simulink model "simple"  (Simulink 7.3)
settings: Solver=ode45  StartTime=0.0  StopTime=200  RelTol=1e-3
libraries: truetime x1
settings Model: Creator=anton  LastModifiedBy=nmd01  ExtModeAutoUpdateStatusClock=off
settings OptimizationCC: BooleanDataType=off
settings DebuggingCC: SaveWithParameterizedLinksMsg=none  SignalResolutionControl=TryResolveAllWithWarning  SolverPrmCheckMsg=none  MultiTaskDSMMsg=warning  MultiTaskCondExecSysMsg=none  StrictBusMsg=None
settings HardwareCC: TargetUnknown=on
settings RTWCC: IncludeERTFirstTime=on

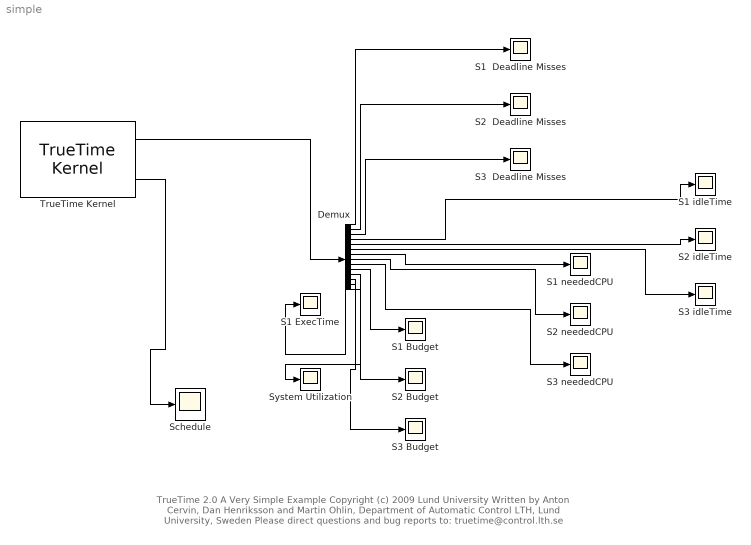
== system simple ==
  note: TrueTime 2.0  A Very Simple Example
      | Copyright (c) 2009 Lund University
      | Written by Anton Cervin, Dan Henriksson and Martin Ohlin,
      | Department of Automatic Control LTH, Lund University, Sweden
      | Please direct questions and bug reports to: truetime@control.lth.se
  Demux : Demux  Outputs=14
  S1 Budget : Scope
      settings: TimeRange=10  YMin=0  YMax=2  SaveName=ScopeData10
  S1 ExecTime : Scope
      settings: TimeRange=10  YMin=0  YMax=2  SaveName=ScopeData13
  S1 idleTime : Scope
      settings: TimeRange=10  YMin=0  YMax=2  SaveName=ScopeData4
  S1 neededCPU : Scope
      settings: TimeRange=10  YMin=0  YMax=2  SaveName=ScopeData7
  S1  Deadline Misses : Scope
      settings: TimeRange=10  YMin=0  YMax=2
  S2 Budget : Scope
      settings: TimeRange=10  YMin=0  YMax=2  SaveName=ScopeData11
  S2 idleTime : Scope
      settings: TimeRange=1000  YMin=0  YMax=0.35  SaveName=ScopeData5
  S2 neededCPU : Scope
      settings: TimeRange=10  YMin=0  YMax=2  SaveName=ScopeData8
  S2  Deadline Misses : Scope
      settings: TimeRange=10  YMin=0  YMax=2  SaveName=ScopeData2
  S3 Budget : Scope
      settings: TimeRange=10  YMin=0  YMax=2  SaveName=ScopeData12
  S3 idleTime : Scope
      settings: TimeRange=10  YMin=0  YMax=2  SaveName=ScopeData6
  S3 neededCPU : Scope
      settings: TimeRange=10  YMin=0  YMax=2  SaveName=ScopeData9
  S3  Deadline Misses : Scope
      settings: TimeRange=10  YMin=0  YMax=2  SaveName=ScopeData3
  Schedule : Scope
      settings: TimeRange=10  YMin=1  YMax=20
  System Utilization : Scope
      settings: TimeRange=10  YMin=0.945  YMax=1.06  SaveName=ScopeData14
  TrueTime Kernel : truetime/TrueTime Kernel  SystemSampleTime=-1  sfun=simple_init  args=[]  ninputsoutputs=[0 14]  ntriggers=0  trigtype=falling  nwnodenbr=[]  clockoffsetdrift=[0 0]  schedoutput=on  battery=off  poweroutput=off
  wires:
  TrueTime Kernel/2 -> Schedule/1
  TrueTime Kernel/1 -> Demux/1
  Demux/1 -> S1  Deadline Misses/1
  Demux/2 -> S2  Deadline Misses/1
  Demux/3 -> S3  Deadline Misses/1
  Demux/4 -> S1 idleTime/1
  Demux/5 -> S2 idleTime/1
  Demux/6 -> S3 idleTime/1
  Demux/7 -> S1 neededCPU/1
  Demux/8 -> S2 neededCPU/1
  Demux/9 -> S3 neededCPU/1
  Demux/10 -> S1 Budget/1
  Demux/11 -> S2 Budget/1
  Demux/12 -> S3 Budget/1
  Demux/13 -> S1 ExecTime/1
  Demux/14 -> System Utilization/1
